simulink library "bh_cv_car_drc_library"  (R2017b)
settings: Solver=VariableStepAuto  StartTime=0.0  StopTime=10.0  RelTol=1e-3
undefined symbols (not defined in the file): veh
settings Model: Creator=bhorton  LastModifiedBy=bhorton

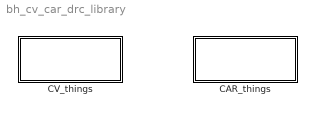
== system bh_cv_car_drc_library ==
  CAR_things : Subsystem
  CV_things : Subsystem

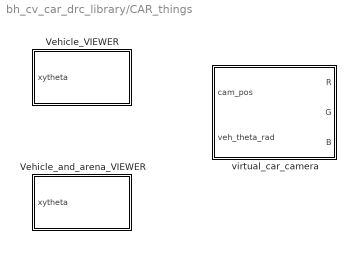
== system bh_cv_car_drc_library/CAR_things ==
  Vehicle_VIEWER : Subsystem  mask{wp_mat=[-1, -1; 2,2], veh_ID_num=1, veh_init_xytheta=[0,0,0], Ts=0.1}
      mask prompts: wp_mat "Waypoint matrix for arena [x_col, y_col] (m)"; veh_ID_num "Vehicle ID number"; veh_init_xytheta "Initial pose [x,y,theta]"; Ts "Sample time for updating animation (secs)"
      mask TypeOptions veh_ID_num: 1 | 2 | 3 | 4
      mask DialogControl Control2 Prompt: Animate simulation of 4Wheel, 3-dof car model
      mask Display: fprintf('veh_ID=%d \n\n 4-wheel, 3-dof',veh_ID_num);
  Vehicle_and_arena_VIEWER : Subsystem  mask{veh_ID_num=1, veh_init_xytheta=veh.states.init_pose, Ts=0.2}
      mask prompts: veh_ID_num "Vehicle ID number"; veh_init_xytheta "Initial pose [x,y,theta]"; Ts "Sample time for updating animation (secs)"
      mask TypeOptions veh_ID_num: 1 | 2 | 3 | 4
      mask DialogControl Control2 Prompt: Animate simulation of 4Wheel, 3-dof car model
      mask Display: fprintf('veh_ID=%d \n\n 4-wheel, 3-dof',veh_ID_num);
  virtual_car_camera : Subsystem  mask(BH_VIRTUAL_CAR_CAMERA){obstacle_visibility=SHOW_OBSTACLES, W=320, H=240, Ts=0.1, init_cam_pos_wrt_W=[0,0], height_of_cam=0.4, init_veh_THETA_wrt_W=0, horz_look_dist=100, cam_va=11}
      mask prompts: obstacle_visibility "Obstacle presence"; W "Pixel WIDTH"; H "Pixel HEIGHT"; Ts "Sample Time (secs)"; init_cam_pos_wrt_W "Initial camera position (xy) rel to WORLD frame"; height_of_cam "Height of camera wrt VEHICLE frame (m)"; init_veh_THETA_wrt_W "Initial vehicle THETA wrt WORLD frame (rads)"; horz_look_dist "Horizontal look ahead distance (m)"; cam_va "Camera View Angle (degrees)"
      mask help:
      | This is a VIRTUAL camera used for testing a VISION based control law for our 4wheel, 3-dof car model
      |
      | BLOCK input ports:
      |    1.) Camera Position  (x,y),  1_x_2, DOUBLE
      |    2.) Vehicle THETA (radians) with respect to WORLD Frame,   scalar DOUBLE
      |
      | BLOCK output ports:
      |    1.) R   I  (with matrix size:   H_x_W ) and UINT8
      |    2.) G   I  (with matrix size:   H_x_W ) and UINT8
      |    3.) B   I  (with matrix size:   H_x_W ) and UINT8
      mask init:
      | tf_obstacles_are_visible = false;
      | if(strcmp(obstacle_visibility,'SHOW_OBSTACLES'))
      |     tf_obstacles_are_visible = true;
      | end
      | 
      | fprintf('\n #### obstacle_visibility     --->  %s ',obstacle_visibility);
      | fprintf('\n #### tf_obstacles_are_visible ---> %d ',tf_obstacles_are_visible);
      mask TypeOptions obstacle_visibility: SHOW_OBSTACLES | HIDE_OBSTACLES
      mask DialogControl Container12 Prompt: TRACK Configuration
      mask DialogControl Control2 Prompt: a Place Holder - currently there is only 1 track
      mask DialogControl Container5 Prompt: CAMERA params
      mask DialogControl Container6 Prompt: CAMERA position
      mask DialogControl Control3 Prompt: The camera view angle determines the field of view of the camera. Larger angles produce a smaller view of the scene. Implement zooming by changing the camera view angle.
      mask Display: disp('VIRTUAL\nCar\nCamera')

== system bh_cv_car_drc_library/CV_things ==

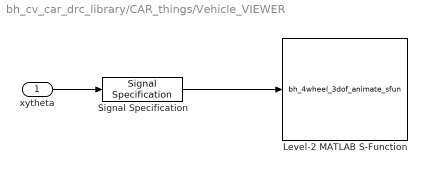
== system bh_cv_car_drc_library/CAR_things/Vehicle_VIEWER ==
  xytheta : Inport
  Level-2 MATLAB S-Function : M-S-Function  FunctionName=bh_4wheel_3dof_animate_sfun  Parameters=Ts, wp_mat, veh_ID_num, veh_init_xytheta
  Signal Specification : SignalSpecification  Dimensions=3
  wires:
  xytheta/1 -> Signal Specification/1
  Signal Specification/1 -> Level-2 MATLAB S-Function/1

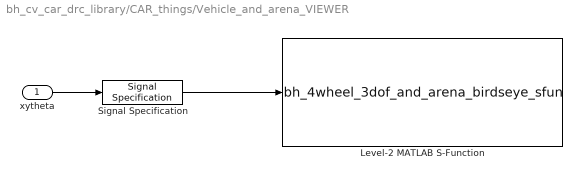
== system bh_cv_car_drc_library/CAR_things/Vehicle_and_arena_VIEWER ==
  xytheta : Inport
  Level-2 MATLAB S-Function : M-S-Function  FunctionName=bh_4wheel_3dof_and_arena_birdseye_sfun  Parameters=Ts, veh_ID_num, veh_init_xytheta
  Signal Specification : SignalSpecification  Dimensions=3
  wires:
  Signal Specification/1 -> Level-2 MATLAB S-Function/1
  xytheta/1 -> Signal Specification/1

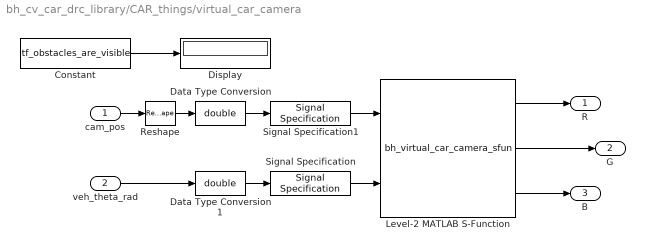
== system bh_cv_car_drc_library/CAR_things/virtual_car_camera ==
  cam_pos : Inport
  veh_theta_rad : Inport  Port=2
  Constant : Constant  Value=tf_obstacles_are_visible
  Data Type Conversion : DataTypeConversion  OutDataTypeStr=double
  Data Type Conversion1 : DataTypeConversion  OutDataTypeStr=double
  Display : Display
  Level-2 MATLAB S-Function : M-S-Function  FunctionName=bh_virtual_car_camera_sfun  Parameters=init_cam_pos_wrt_W,init_veh_THETA_wrt_W, height_of_cam, horz_look_dist,W,H,Ts,cam_va,tf_obstacles_are_visible
  Reshape : Reshape  OutputDimensionality=Row vector (2-D)
  Signal Specification : SignalSpecification  OutDataTypeStr=double  Dimensions=[1 1]
  Signal Specification1 : SignalSpecification  OutDataTypeStr=double  Dimensions=[1 2]
  R : Outport
  G : Outport  Port=2
  B : Outport  Port=3
  wires:
  Constant/1 -> Display/1
  cam_pos/1 -> Reshape/1
  Level-2 MATLAB S-Function/1 -> R/1
  veh_theta_rad/1 -> Data Type Conversion1/1
  Level-2 MATLAB S-Function/2 -> G/1
  Level-2 MATLAB S-Function/3 -> B/1
  Reshape/1 -> Data Type Conversion/1
  Data Type Conversion/1 -> Signal Specification1/1
  Data Type Conversion1/1 -> Signal Specification/1
  Signal Specification/1 -> Level-2 MATLAB S-Function/2
  Signal Specification1/1 -> Level-2 MATLAB S-Function/1
